simulink model "omnimorph_controller_FL"  (R2023b)
settings: Solver=ode1  StartTime=0.0  StopTime=inf  FixedStep=config.simVar.timeStep  RelTol=1e-3
libraries: genomix x5, robotcorelib x4
settings Model: Creator=amr  LastModifiedBy=fiore
settings DataIOCC: ReturnWorkspaceOutputs=off
settings OptimizationCC: ReuseModelBlockBuffer=off
settings DebuggingCC: UnconnectedInputMsg=warning  UnconnectedOutputMsg=warning  UnconnectedLineMsg=warning  UnderSpecifiedDimensionMsg=warning
settings ModelReferenceCC: EnableRefExpFcnMdlSchedulingChecks=on
settings RTWCC: DLArmComputeVersion=19.05

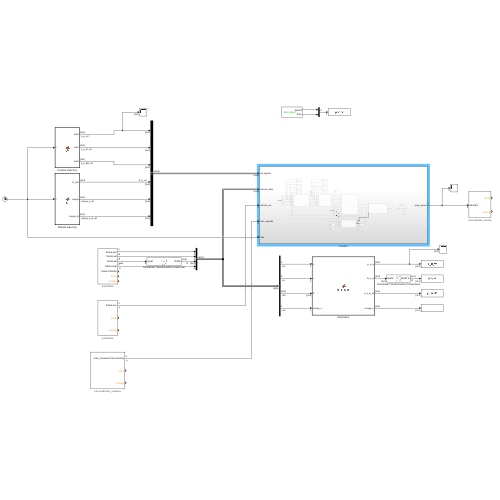
[thumbnail: Simulink's stored preview of the top-level diagram]
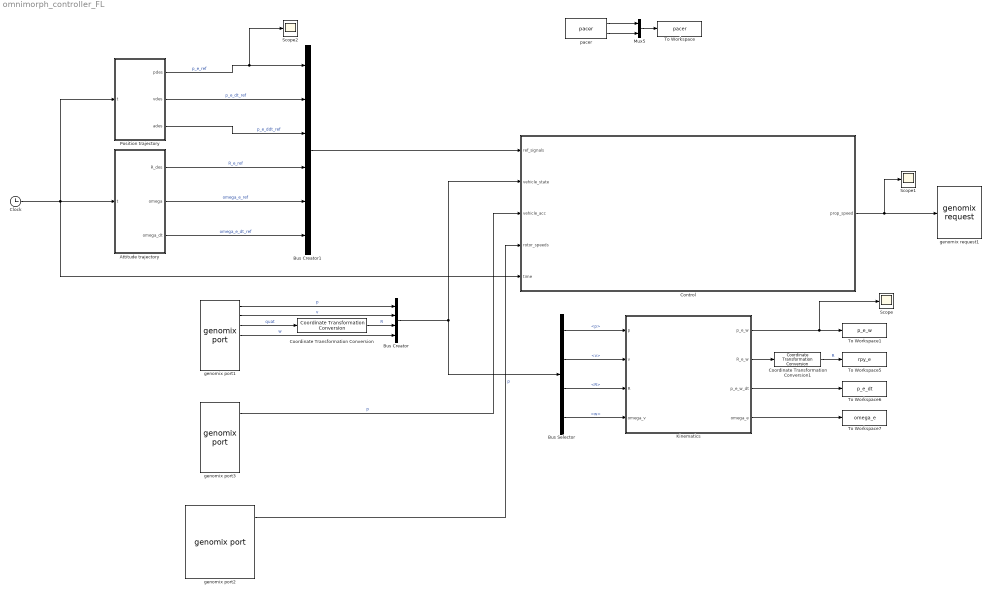
== system omnimorph_controller_FL ==
  Attitude trajectory : MATLAB Function  TreatAsAtomicUnit=on
  Bus Creator : BusCreator  Inputs=4
  Bus Creator1 : BusCreator  Inputs=6
  Bus Selector : BusSelector  OutputSignals=p,v,R,w
  Clock : Clock
  Control : Subsystem
  Coordinate Transformation Conversion : robotcorelib/Coordinate Transformation Conversion  InputRepresentation=Quaternion  InputEulerSequence=ZYX  ShowTrVecInputPort=on  OutputRepresentation=Rotation Matrix  OutputEulerSequence=ZYX  ShowTrVecOutputPort=on  SimulateUsing=Interpreted execution
  Coordinate Transformation Conversion1 : robotcorelib/Coordinate Transformation Conversion  InputRepresentation=Rotation Matrix  InputEulerSequence=ZYX  ShowTrVecInputPort=on  OutputRepresentation=Euler Angles  OutputEulerSequence=ZYX  ShowTrVecOutputPort=on  SimulateUsing=Interpreted execution
  Kinematics : MATLAB Function  TreatAsAtomicUnit=on
  Mux5 : Mux  Inputs=2
  Position trajectory : MATLAB Function  TreatAsAtomicUnit=on
  Scope : Scope
  Scope1 : Scope
  Scope2 : Scope
  To Workspace : ToWorkspace  VariableName=pacer  SaveFormat=Timeseries  SampleTime=-1
  To Workspace1 : ToWorkspace  VariableName=p_e_w  SampleTime=-1
  To Workspace5 : ToWorkspace  VariableName=rpy_e  SampleTime=-1
  To Workspace6 : ToWorkspace  VariableName=p_e_dt  SampleTime=-1
  To Workspace7 : ToWorkspace  VariableName=omega_e  SampleTime=-1
  genomix port1 : genomix/genomix port  host=localhost  component=pom  port=frame  subport=robot  sigtype=value  timetype=periodic  period=config.simVar.timeStep  siglist="[{\"name\":\"frame.pos\",\"type\":\"value\",\"size\":3},{\"name\":\"frame.vel\",\"type\":\"value\",\"size\":3},{\"name\":\"frame.att\",\"type\":\"value\",\"size\":4},{\"name\":\"frame.avel\",\"type\":\"value\",\"size\":3},{\"name\":\"frame.intrinsic\",\"type\":\"value\",\"size\":1}]"
      settings: AttributesFormatString=pom/frame
  genomix port2 : genomix/genomix port  host=localhost  component=rotorcraft  port=rotor_measure  sigtype=value  timetype=periodic  period=config.simVar.timeStep  siglist="[{\"name\":\"rotor_measure.rotor.velocity\",\"type\":\"value\",\"size\":8}]"
      settings: AttributesFormatString=rotorcraft/rotor_measure
  genomix port3 : genomix/genomix port  host=localhost  component=pom  port=frame  subport=robot  sigtype=value  timetype=periodic  period=config.simVar.timeStep  siglist="[{\"name\":\"frame.acc\",\"type\":\"value\",\"size\":3}]"
      settings: AttributesFormatString=pom/frame
  genomix request1 : genomix/genomix request  host=localhost  component=rotorcraft  port=set_velocity  sigtype=value  timetype=periodic  period=config.simVar.timeStep  siglist="[{\"name\":\"desired\",\"type\":\"value\",\"size\":8}]"
      settings: AttributesFormatString=rotorcraft/set_velocity
  pacer : genomix/pacer  Priority=0  catchup=off
  wires:
  genomix port1/1 -> Bus Creator/1  "p"
  genomix port1/2 -> Bus Creator/2  "v"
  genomix port1/4 -> Bus Creator/4  "w"
  genomix port1/3 -> Coordinate Transformation Conversion/1  "quat"
  Coordinate Transformation Conversion/1 -> Bus Creator/3  "R"
  Bus Creator/1 -> Bus Selector/1, Control/2(vehicle_state)
  Control/1(prop_speed) -> Scope1/1, genomix request1/1
  pacer/2 -> Mux5/2
  pacer/1 -> Mux5/1
  Mux5/1 -> To Workspace/1
  genomix port3/1 -> Control/3(vehicle_acc)  "p"
  genomix port2/1 -> Control/4(rotor_speeds)  "p"
  Kinematics/1(p_e_w) -> Scope/1, To Workspace1/1
  Kinematics/3(p_e_w_dt) -> To Workspace6/1
  Kinematics/4(omega_e) -> To Workspace7/1
  Coordinate Transformation Conversion1/1 -> To Workspace5/1  "R"
  Kinematics/2(R_e_w) -> Coordinate Transformation Conversion1/1
  Bus Selector/1 -> Kinematics/1(p)  "<p>"
  Bus Selector/2 -> Kinematics/2(v)  "<v>"
  Bus Selector/3 -> Kinematics/3(R)  "<R>"
  Bus Selector/4 -> Kinematics/4(omega_v)  "<w>"
  Attitude trajectory/1(R_des) -> Bus Creator1/4  "R_e_ref"
  Attitude trajectory/2(omega) -> Bus Creator1/5  "omega_e_ref"
  Position trajectory/3(ades) -> Bus Creator1/3  "p_e_ddt_ref"
  Clock/1 -> Control/5(time), Position trajectory/1(t), Attitude trajectory/1(t)
  Bus Creator1/1 -> Control/1(ref_signals)
  Position trajectory/2(vdes) -> Bus Creator1/2  "p_e_dt_ref"
  Attitude trajectory/3(omega_dt) -> Bus Creator1/6  "omega_e_dt_ref"
  Position trajectory/1(pdes) -> Scope2/1, Bus Creator1/1  "p_e_ref"

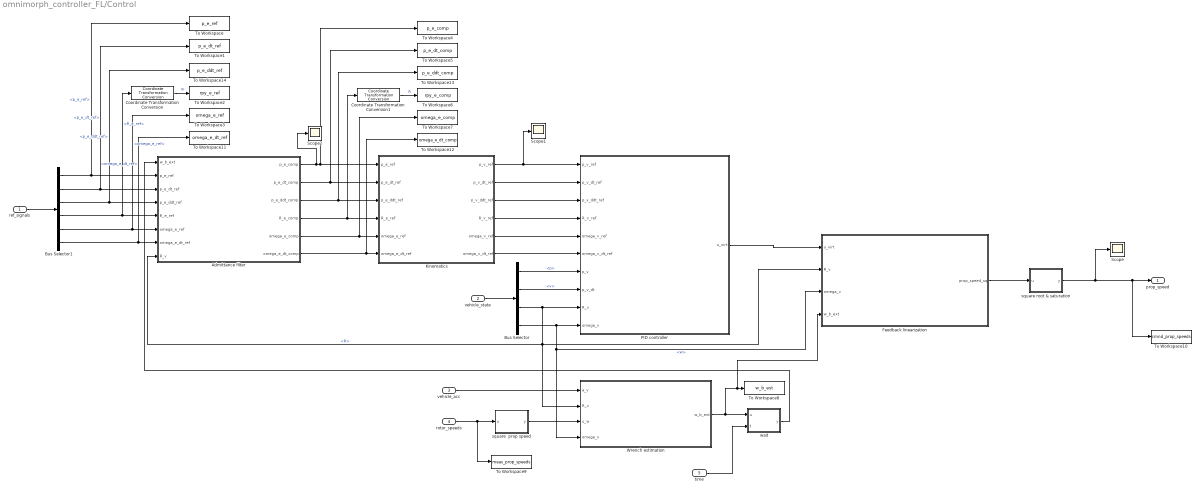
== system omnimorph_controller_FL/Control ==
  ref_signals : Inport
  vehicle_state : Inport  Port=2
  vehicle_acc : Inport  Port=3
  rotor_speeds : Inport  Port=4
  time : Inport  Port=5
  Admittance filter : Subsystem
  Bus Selector : BusSelector  OutputSignals=p,v,R,w
  Bus Selector1 : BusSelector  OutputSignals=p_e_ref,p_e_dt_ref,p_e_ddt_ref,R_e_ref,omega_e_ref,omega_e_dt_ref
  Coordinate Transformation Conversion : robotcorelib/Coordinate Transformation Conversion  InputRepresentation=Rotation Matrix  InputEulerSequence=ZYX  ShowTrVecInputPort=on  OutputRepresentation=Euler Angles  OutputEulerSequence=ZYX  ShowTrVecOutputPort=on  SimulateUsing=Interpreted execution
  Coordinate Transformation Conversion1 : robotcorelib/Coordinate Transformation Conversion  InputRepresentation=Rotation Matrix  InputEulerSequence=ZYX  ShowTrVecInputPort=on  OutputRepresentation=Euler Angles  OutputEulerSequence=ZYX  ShowTrVecOutputPort=on  SimulateUsing=Interpreted execution
  Feedback linearization : MATLAB Function  TreatAsAtomicUnit=on
  Kinematics : MATLAB Function  TreatAsAtomicUnit=on
  PID controller : MATLAB Function  TreatAsAtomicUnit=on
  Scope : Scope
  Scope1 : Scope
  Scope2 : Scope
  To Workspace : ToWorkspace  VariableName=p_e_ref  SampleTime=-1
  To Workspace1 : ToWorkspace  VariableName=p_e_dt_ref  SampleTime=-1
  To Workspace10 : ToWorkspace  VariableName=cmnd_prop_speeds  SampleTime=-1
  To Workspace11 : ToWorkspace  VariableName=omega_e_dt_ref  SampleTime=-1
  To Workspace12 : ToWorkspace  VariableName=omega_e_dt_comp  SampleTime=-1
  To Workspace13 : ToWorkspace  VariableName=p_e_ddt_comp  SampleTime=-1
  To Workspace14 : ToWorkspace  VariableName=p_e_ddt_ref  SampleTime=-1
  To Workspace2 : ToWorkspace  VariableName=rpy_e_ref  SampleTime=-1
  To Workspace3 : ToWorkspace  VariableName=omega_e_ref  SampleTime=-1
  To Workspace4 : ToWorkspace  VariableName=p_e_comp  SampleTime=-1
  To Workspace5 : ToWorkspace  VariableName=p_e_dt_comp  SampleTime=-1
  To Workspace6 : ToWorkspace  VariableName=rpy_e_comp  SampleTime=-1
  To Workspace7 : ToWorkspace  VariableName=omega_e_comp  SampleTime=-1
  To Workspace8 : ToWorkspace  VariableName=w_b_est  SampleTime=-1
  To Workspace9 : ToWorkspace  VariableName=meas_prop_speeds  SampleTime=-1
  Wrench estimation : Subsystem
  square  prop speed : MATLAB Function  TreatAsAtomicUnit=on
  square root & saturation : MATLAB Function  TreatAsAtomicUnit=on
  wait : MATLAB Function  TreatAsAtomicUnit=on
  prop_speed : Outport
  wires:
  PID controller/1(u_virt) -> Feedback linearization/1(u_virt)
  Bus Selector/4 -> PID controller/10(omega_v), Wrench estimation/4(omega_v), Feedback linearization/3(omega_v)  "<w>"
  ref_signals/1 -> Bus Selector1/1
  square root & saturation/1(y) -> Scope/1, prop_speed/1, To Workspace10/1
  Admittance filter/1(p_e_comp) -> Scope2/1, To Workspace4/1, Kinematics/1(p_e_ref)
  Admittance filter/2(p_e_dt_comp) -> To Workspace5/1, Kinematics/2(p_e_dt_ref)
  Admittance filter/3(p_e_ddt_comp) -> To Workspace13/1, Kinematics/3(p_e_ddt_ref)
  Admittance filter/6(omega_e_dt_comp) -> To Workspace12/1, Kinematics/6(omega_e_dt_ref)
  Bus Selector1/6 -> To Workspace11/1, Admittance filter/7(omega_e_dt_ref)  "<omega_e_dt_ref>"
  Bus Selector1/5 -> To Workspace3/1, Admittance filter/6(omega_e_ref)  "<omega_e_ref>"
  Bus Selector1/4 -> Admittance filter/5(R_e_ref), Coordinate Transformation Conversion/1  "<R_e_ref>"
  Bus Selector1/3 -> To Workspace14/1, Admittance filter/4(p_e_ddt_ref)  "<p_e_ddt_ref>"
  Bus Selector1/2 -> To Workspace1/1, Admittance filter/3(p_e_dt_ref)  "<p_e_dt_ref>"
  Admittance filter/4(R_e_comp) -> Kinematics/4(R_e_ref), Coordinate Transformation Conversion1/1
  Kinematics/1(p_v_ref) -> Scope1/1, PID controller/1(p_v_ref)
  Kinematics/2(p_v_dt_ref) -> PID controller/2(p_v_dt_ref)
  Kinematics/3(p_v_ddt_ref) -> PID controller/3(p_v_ddt_ref)
  Kinematics/5(omega_v_ref) -> PID controller/5(omega_v_ref)
  Kinematics/6(omega_v_dt_ref) -> PID controller/6(omega_v_dt_ref)
  Kinematics/4(R_v_ref) -> PID controller/4(R_v_ref)
  Admittance filter/5(omega_e_comp) -> Kinematics/5(omega_e_ref), To Workspace7/1
  Bus Selector/1 -> PID controller/7(p_v)  "<p>"
  Bus Selector/2 -> PID controller/8(p_v_dt)  "<v>"
  Bus Selector/3 -> Wrench estimation/2(R_v), Admittance filter/8(R_v), Feedback linearization/2(R_v), PID controller/9(R_v)  "<R>"
  Feedback linearization/1(prop_speed_sq) -> square root & saturation/1(u)
  vehicle_state/1 -> Bus Selector/1
  vehicle_acc/1 -> Wrench estimation/1(a_v)
  rotor_speeds/1 -> To Workspace9/1, square  prop speed/1(u)
  square  prop speed/1(y) -> Wrench estimation/3(u_w)
  wait/1(y) -> Admittance filter/1(w_b_ext)
  time/1 -> wait/2(t)
  Bus Selector1/1 -> To Workspace/1, Admittance filter/2(p_e_ref)  "<p_e_ref>"
  Wrench estimation/1(w_b_ext) -> Feedback linearization/4(w_b_ext), To Workspace8/1, wait/1(u)
  Coordinate Transformation Conversion/1 -> To Workspace2/1  "R"
  Coordinate Transformation Conversion1/1 -> To Workspace6/1  "R"

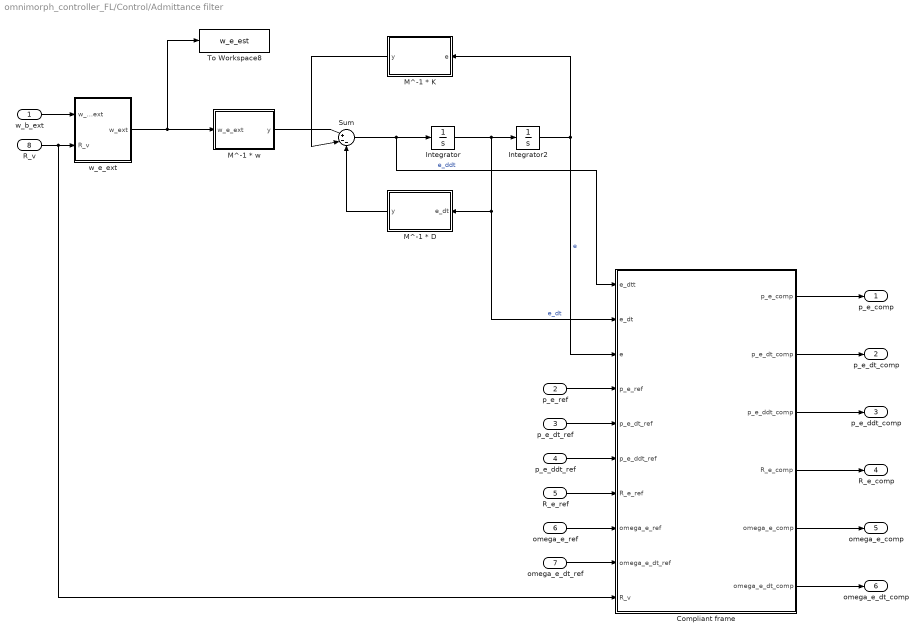
== system omnimorph_controller_FL/Control/Admittance filter ==
  w_b_ext : Inport
  p_e_ref : Inport  Port=2
  p_e_dt_ref : Inport  Port=3
  p_e_ddt_ref : Inport  Port=4
  R_e_ref : Inport  Port=5
  omega_e_ref : Inport  Port=6
  omega_e_dt_ref : Inport  Port=7
  R_v : Inport  Port=8
  Compliant frame : MATLAB Function  TreatAsAtomicUnit=on
  Integrator : Integrator
  Integrator2 : Integrator
  M^-1 * D : MATLAB Function  TreatAsAtomicUnit=on
  M^-1 * K : MATLAB Function  TreatAsAtomicUnit=on
  M^-1 * w : MATLAB Function  TreatAsAtomicUnit=on
  Sum : Sum  Inputs=|+--
  To Workspace8 : ToWorkspace  VariableName=w_e_est  SampleTime=-1
  w_e_ext : MATLAB Function  TreatAsAtomicUnit=on
  p_e_comp : Outport
  p_e_dt_comp : Outport  Port=2
  p_e_ddt_comp : Outport  Port=3
  R_e_comp : Outport  Port=4
  omega_e_comp : Outport  Port=5
  omega_e_dt_comp : Outport  Port=6
  wires:
  Integrator/1 -> Compliant frame/2(e_dt), M^-1 * D/1(e_dt), Integrator2/1  "e_dt"
  Sum/1 -> Compliant frame/1(e_dtt), Integrator/1  "e_ddt"
  M^-1 * K/1(y) -> Sum/2
  Integrator2/1 -> Compliant frame/3(e), M^-1 * K/1(e)  "e"
  M^-1 * D/1(y) -> Sum/3
  p_e_ref/1 -> Compliant frame/4(p_e_ref)
  p_e_dt_ref/1 -> Compliant frame/5(p_e_dt_ref)
  p_e_ddt_ref/1 -> Compliant frame/6(p_e_ddt_ref)
  R_e_ref/1 -> Compliant frame/7(R_e_ref)
  omega_e_ref/1 -> Compliant frame/8(omega_e_ref)
  omega_e_dt_ref/1 -> Compliant frame/9(omega_e_dt_ref)
  Compliant frame/6(omega_e_dt_comp) -> omega_e_dt_comp/1
  Compliant frame/5(omega_e_comp) -> omega_e_comp/1
  Compliant frame/4(R_e_comp) -> R_e_comp/1
  Compliant frame/3(p_e_ddt_comp) -> p_e_ddt_comp/1
  Compliant frame/2(p_e_dt_comp) -> p_e_dt_comp/1
  Compliant frame/1(p_e_comp) -> p_e_comp/1
  M^-1 * w/1(y) -> Sum/1
  w_b_ext/1 -> w_e_ext/1(w_b_ext)
  R_v/1 -> Compliant frame/10(R_v), w_e_ext/2(R_v)
  w_e_ext/1(w_ext) -> To Workspace8/1, M^-1 * w/1(w_e_ext)

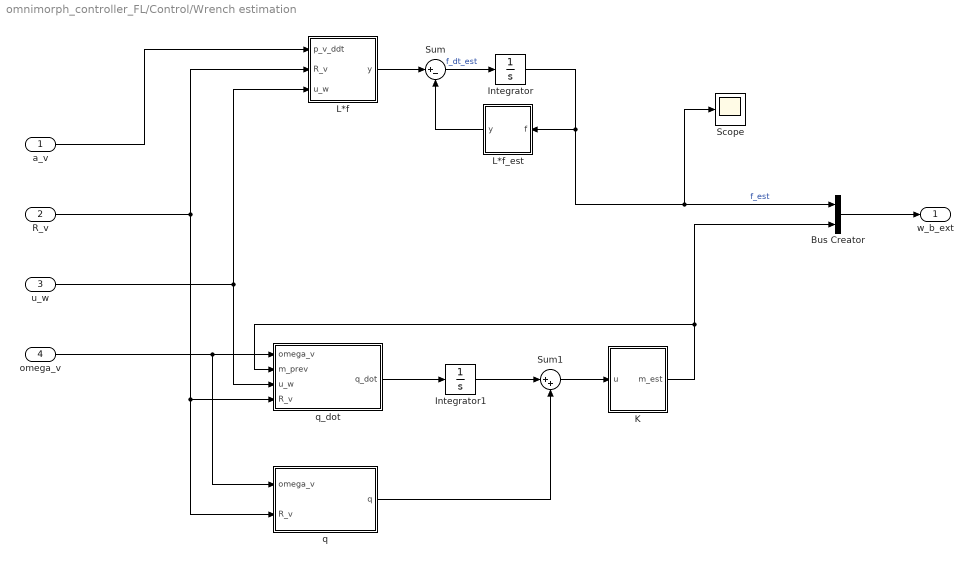
== system omnimorph_controller_FL/Control/Wrench estimation ==
  a_v : Inport
  R_v : Inport  Port=2
  u_w : Inport  Port=3
  omega_v : Inport  Port=4
  Bus Creator : BusCreator  Inputs=2
  Integrator : Integrator
  Integrator1 : Integrator
  K : MATLAB Function  TreatAsAtomicUnit=on
  L*f : MATLAB Function  TreatAsAtomicUnit=on
  L*f_est : MATLAB Function  TreatAsAtomicUnit=on
  Scope : Scope
  Sum : Sum  Inputs=|+-
  Sum1 : Sum  Inputs=|++
  q : MATLAB Function  TreatAsAtomicUnit=on
  q_dot : MATLAB Function  TreatAsAtomicUnit=on
  w_b_ext : Outport
  wires:
  Sum/1 -> Integrator/1  "f_dt_est"
  Integrator/1 -> Scope/1, Bus Creator/1, L*f_est/1(f)  "f_est"
  L*f_est/1(y) -> Sum/2
  L*f/1(y) -> Sum/1
  R_v/1 -> q/2(R_v), q_dot/4(R_v), L*f/2(R_v)
  u_w/1 -> q_dot/3(u_w), L*f/3(u_w)
  omega_v/1 -> q/1(omega_v), q_dot/1(omega_v)
  a_v/1 -> L*f/1(p_v_ddt)
  Integrator1/1 -> Sum1/1
  q/1(q) -> Sum1/2
  Sum1/1 -> K/1(u)
  q_dot/1(q_dot) -> Integrator1/1
  Bus Creator/1 -> w_b_ext/1
  K/1(m_est) -> Bus Creator/2, q_dot/2(m_prev)

== matlab function omnimorph_controller_FL/Control/Admittance filter/M^-1 * D ==
  data: e_dt input; y output; config parameter
function y = fcn(e_dt,config)

D = config.conrtolParams.admitFilt.virtDamp;
M = config.conrtolParams.admitFilt.virtMass;
%invM = diag([1/M(1,1);1/M(2,2);1/M(3,3)]);
invM = diag([1/M(1,1);1/M(2,2);1/M(3,3);1/M(4,4);1/M(5,5);1/M(6,6)]);

y = invM*D*e_dt;

end

== matlab function omnimorph_controller_FL/Control/Admittance filter/Compliant frame ==
  data: e_dtt input; e_dt input; e input; p_e_ref input; p_e_dt_ref input; p_e_ddt_ref input; R_e_ref input; omega_e_ref input; omega_e_dt_ref input; R_v input; p_e_comp output; config parameter; p_e_dt_comp output; p_e_ddt_comp output; R_e_comp output; omega_e_comp output; omega_e_dt_comp output
function [p_e_comp,p_e_dt_comp,p_e_ddt_comp,R_e_comp,omega_e_comp,omega_e_dt_comp] = fcn(e_dtt,e_dt,e,p_e_ref,p_e_dt_ref,p_e_ddt_ref, ...
                                                                                 R_e_ref,omega_e_ref,omega_e_dt_ref,R_v,config)
p_e_comp = p_e_ref + e(1:3);
p_e_dt_comp = p_e_dt_ref + e_dt(1:3);
p_e_ddt_comp = p_e_ddt_ref + e_dtt(1:3);

R_e_comp = (skewMat(e(4:6)) + eye(3))*R_e_ref;
omega_e_comp = omega_e_ref + e_dt(4:6);
omega_e_dt_comp = omega_e_dt_ref + e_dtt(4:6);
end

== matlab function omnimorph_controller_FL/Control/Admittance filter/M^-1 * w ==
  data: w_e_ext input; y output; config parameter
function y = fcn(w_e_ext,config)

M = config.conrtolParams.admitFilt.virtMass;
invM = diag([1/M(1,1);1/M(2,2);1/M(3,3);1/M(4,4);1/M(5,5);1/M(6,6)]);

y = invM*w_e_ext;

end

== matlab function omnimorph_controller_FL/Kinematics ==
  settings: updateMethod=DISCRETE
  data: p input; v input; R input; omega_v input; config parameter; p_e_w output; R_e_w output; p_e_w_dt output; omega_e output
function [p_e_w,R_e_w,p_e_w_dt,omega_e] = kinematic(p,v,R,omega_v,config)

p_e = config.uavParams.endEffector.p_e;
R_e = config.uavParams.endEffector.R_e;

p_e_w = p + R*p_e;
R_e_w = R*R_e;

omega_e = omega_v;
p_e_w_dt = v + R*skewMat(omega_v)*p_e;

end

== matlab function omnimorph_controller_FL/Control/Kinematics ==
  settings: updateMethod=DISCRETE
  data: p_e_ref input; p_e_dt_ref input; p_e_ddt_ref input; R_e_ref input; omega_e_ref input; omega_e_dt_ref input; config parameter; p_v_ref output; p_v_dt_ref output; p_v_ddt_ref output; R_v_ref output; omega_v_ref output; omega_v_dt_ref output
function [p_v_ref,p_v_dt_ref,p_v_ddt_ref,R_v_ref,omega_v_ref,omega_v_dt_ref] = kinematic(p_e_ref,p_e_dt_ref,p_e_ddt_ref,R_e_ref,omega_e_ref,omega_e_dt_ref,config)

p_e = config.uavParams.endEffector.p_e ;
R_e = config.uavParams.endEffector.R_e;

% R_v_ref = R_e_ref*R_e.';
% p_v_ref = p_e_ref - R_v_ref*p_e;
% 
% omega_v_ref = omega_e_ref;
% p_v_dt_ref = p_e_dt_ref - R_v_ref*skewMat(omega_v_ref)*p_e;
% 
% omega_v_dt_ref = omega_e_dt_ref;
% p_v_ddt_ref = p_e_ddt_ref - R_v_ref*skewMat(omega_v_dt_ref)*p_e - R_v_ref*skewMat(omega_v_ref)^2 *p_e;

R_v_ref = R_e_ref*R_e.';
p_v_ref = p_e_ref - R_v_ref*p_e;

omega_v_ref = omega_e_ref;
p_v_dt_ref = p_e_dt_ref - skewMat(omega_v_ref)*R_v_ref*p_e;

omega_v_dt_ref = omega_e_dt_ref;
p_v_ddt_ref = p_e_ddt_ref - skewMat(omega_v_dt_ref)*R_v_ref*p_e - skewMat(omega_v_ref)^2 *R_v_ref*p_e;
end

== matlab function omnimorph_controller_FL/Control/Wrench estimation/L*f_est ==
  settings: updateMethod=DISCRETE
  data: f input; config parameter; y output
function y = fcn(f,config)

L = config.conrtolParams.wrenchObs.gains(1:3,1:3);
y = L*f;

end

== matlab function omnimorph_controller_FL/Control/Wrench estimation/L*f ==
  settings: updateMethod=DISCRETE
  data: p_v_ddt input; R_v input; u_w input; config parameter; y output
function y = fcn(p_v_ddt,R_v,u_w,config)

L = config.conrtolParams.wrenchObs.gains(1:3,1:3);
m = config.uavParams.mass;
g = config.gravity;
A = config.uavParams.wrenchMap;

f = m*p_v_ddt + m*g*[0;0;1] - R_v*A(1:3,:)*u_w;

y = L*f;

end

== matlab function omnimorph_controller_FL/Control/Wrench estimation/q_dot ==
  settings: updateMethod=DISCRETE
  data: omega_v input; m_prev input; u_w input; R_v input; config parameter; q_dot output size=[3 1]
function q_dot = fcn(omega_v,m_prev,u_w,R_v,config)

A = config.uavParams.wrenchMap;
J = config.uavParams.inertia;
omega_v_b = R_v'*omega_v; % Body frame angular velocity

q_dot = cross(omega_v_b,(J*omega_v_b)) - A(4:6,:)*u_w - m_prev;

end

== matlab function omnimorph_controller_FL/Control/Wrench estimation/q ==
  settings: updateMethod=DISCRETE
  data: omega_v input; R_v input; config parameter; q output
function q = fcn(omega_v,R_v,config)

J = config.uavParams.inertia;
omega_v_b = R_v'*omega_v; % Body frame angular velocity

% Assuming initial angular velocity is zero
q = J*omega_v_b;

end

== matlab function omnimorph_controller_FL/Control/Wrench estimation/K ==
  settings: updateMethod=DISCRETE
  data: u input; config parameter; m_est output
function m_est = fcn(u,config)

K = config.conrtolParams.wrenchObs.gains(4:6,4:6);
m_est = K*u;

end

== matlab function omnimorph_controller_FL/Control/Admittance filter/w_e_ext ==
  data: w_b_ext input; R_v input; w_ext output; config parameter
function w_ext = fcn(w_b_ext,R_v,config)

p_e = config.uavParams.endEffector.p_e;

H =  [eye(3),zeros(3);skewMat(R_v*p_e),eye(3)];
w_ext = H\[w_b_ext(1:3);R_v*w_b_ext(4:6)];

end

== matlab function omnimorph_controller_FL/Control/square root & saturation ==
  data: u input; y output; config parameter
function y = fcn(u,config)   
    prop_max = config.uavParams.maxPropSpeed;
    prop_min = config.uavParams.minPropSpeed;

    y = sign(u) .* sqrt(abs(u));
    y = min(y, prop_max); % Clip positive values
    y = max(y, prop_min); % Clip negative values
end

== matlab function omnimorph_controller_FL/Position trajectory ==
  data: t input; pdes output; vdes output; ades output; config parameter
function [pdes,vdes,ades] = fcn(t,config)

r = config.trajParams.radius;
f = config.trajParams.frequency;
z = 1;

% Circular trajectory
if t<2
   [pdes,vdes,ades] = circ_traj(t,0.5*t,f,0.5*t);
   vdes(3) = 0.5;
else
   [pdes,vdes,ades] = circ_traj(t,r,f,z);
end

% Peg-in-hole task
% if t<2
%     pdes = [0;0;0.5*t];
%     vdes = [0;0;0.5];
%     ades = [0;0;0];
% elseif t>=2 && t<16.5
%     pdes = [0.1*(t-2);0;0.99];
%     vdes = [0.1;0;0];
%     ades = [0;0;0];
% else
%     pdes = [(0.1*(16.5-2))-0.1*(t-16.5);0;0.99];
%     vdes = [-0.1;0;0];
%     ades = [0;0;0];    
% end

% Sliding task
%if t<2
%    pdes = [0;0;0.5*t];
%    vdes = [0;0;0.5];
%    ades = [0;0;0];
%elseif t>=2 && t<14
%   pdes = [0.1*(t-2);0;1];
%   vdes = [0.1;0;0];
%   ades = [0;0;0]; 
%else
%   pdes = [1.2;0;1+0.1*(t-14)];
%   vdes = [0;0;0.1];
%   ades = [0;0;0]; 
%end

end

== matlab function omnimorph_controller_FL/Control/PID controller ==
  settings: updateMethod=DISCRETE
  data: p_v_ref input; p_v_dt_ref input; p_v_ddt_ref input; R_v_ref input; omega_v_ref input; omega_v_dt_ref input; p_v input; p_v_dt input; R_v input; omega_v input; config parameter; u_virt output
function u_virt  = PIDPlus(p_v_ref,p_v_dt_ref,p_v_ddt_ref, ...
                                          R_v_ref,omega_v_ref,omega_v_dt_ref,...
                                          p_v,p_v_dt,...
                                          R_v,omega_v,config)

persistent eI_prev

if isempty(eI_prev)
    eI_prev = zeros(6,1);
end

%% initializations
u_virt = zeros(6,1);

Kp = config.conrtolParams.gainsPID.Kp;
Kv = config.conrtolParams.gainsPID.Kv;
KR = config.conrtolParams.gainsPID.KR;
Kw = config.conrtolParams.gainsPID.Kw;
KI_p = config.conrtolParams.gainsPID.KI_p;

dt = config.simVar.timeStep;

%omega_v = R_v'*omega_v;

%% error signal computations 
ep =  p_v_ref - p_v;
ev = p_v_dt_ref - p_v_dt;
eI_p = eI_prev(1:3) + ep*dt;

eR = vmap(R_v_ref,R_v);
%ew = R_v.' * (omega_v_ref - omega_v);

ew = omega_v_ref - (R_v.')*R_v_ref*omega_v;
eI_R = eI_prev(4:6) + eR*dt;

eI_prev = [eI_p; eI_R];

%% compute u_virt
u_virt(1:3) = p_v_ddt_ref + Kv*ev + Kp*ep + KI_p*eI_p; 
u_virt(4:6) = omega_v_dt_ref + Kw*ew + KR*eR; 
end

== matlab function omnimorph_controller_FL/Control/Feedback linearization ==
  settings: updateMethod=DISCRETE
  data: u_virt input size=[6, 1]; prop_speed_sq output size=[8,1]; R_v input size=[3, 3]; omega_v input; w_b_ext input; config parameter
function prop_speed_sq = cntrl_FL(u_virt,R_v,omega_v,w_b_ext,config)

% initializations
m = config.uavParams.mass; % uav mass
J = config.uavParams.inertia;%3x3 diag. uav Inertia mat.
A = config.uavParams.wrenchMap;
g = config.gravity;
omega_v = R_v'*omega_v;% Body frame angular velocity

J_inv = diag([1/J(1,1),1/J(2,2),1/J(3,3)]);
invInertia_mat = [eye(3)*(1/m), zeros(3); zeros(3),J_inv];
A_bar = invInertia_mat*[R_v, zeros(3); zeros(3), eye(3)]*A;
bias_forces = -[g*[0;0;1];J_inv*cross(omega_v,(J*omega_v))];
w_b = invInertia_mat*w_b_ext;

% feedback linearization
prop_speed_sq = pinv(A_bar)*( - bias_forces + u_virt - w_b);

end

% function prop_speed_sq = cntrl_FL(u_virt,R_v,omega_v,config,t,w_cur)
% % initializations
% m = config.uavParams.mass; % uav mass
% J = config.uavParams.inertia;%3x3 diag. uav Inertia mat.
% A = config.uavParams.wrenchMap;
% g = config.gravity;
% omega_v = R_v'*omega_v;
% J_inv = diag([1/J(1,1),1/J(2,2),1/J(3,3)]);
% invInertia_mat = [eye(3)*(1/m), zeros(3); zeros(3),J_inv];
% A_bar = invInertia_mat*[R_v, zeros(3); zeros(3), eye(3)]*A;
% bias_forces = -[g*[0;0;1];J_inv*cross(omega_v,(J*omega_v))];
% 
% % feedback linearization
% %prop_speed_sq = wrench2u_hybrid(A_bar, (-bias_forces + u_virt), 8);
% 
% lb=30*30; ub=220*220;
% prop_speed_sq = zeros(8,1);  % force fixed size
% 
% persistent y_prev u_prev t_miqp k_miqp y_prev_measured
% 
% if isempty(y_prev)
%     y_prev = ones(8,1);   
% else
%     y_prev = y_prev(:); 
% end
% if isempty(u_prev)
%     u_prev = 50*ones(8,1);
% else
%     u_prev = u_prev(:);
% end
% if isempty(y_prev_measured)
%     y_prev_measured = double(sign(w_cur) > 0);   
% else
%     y_prev_measured = y_prev_measured(:);
% end
% if isempty(t_miqp)
%     t_miqp = 0;  
% end
% if isempty(k_miqp)
%     k_miqp = 0;   
% end
% w_cur_zero_idx=find(w_cur==0);
% y_measured=[];
% if isempty(w_cur_zero_idx)
%     y_measured=double(sign(w_cur) > 0);
% else
%     y_measured=double(sign(w_cur) > 0);
%     y_measured(w_cur_zero_idx)=y_prev_measured(w_cur_zero_idx);
% end
%  y_prev_measured(:)=y_measured;
%  u_pinv = pinv(A_bar)*(-bias_forces + u_virt);
%  pinv_feasible = all(abs(u_pinv) >= lb & abs(u_pinv) <= ub);
%  near_lb_idx = find(y_prev~=y_prev_measured);
%  all_measu=all(y_prev==y_prev_measured & abs(w_cur) >= lb);
%  Q=eye(8,8);
%  w=(-bias_forces + u_virt);
%  A=A_bar;
%  if pinv_feasible && all_measu
%      % Directly accept the pseudoinverse solution
%      prop_speed_sq(:) = u_pinv(:);
%      u_prev(:) = u_pinv(:);
%      sgn = sign(u_pinv);
%      y_prev = double(sgn > 0);
%  else
%      tic;
%      % --- Identify indices near lower bound ---
%      if ~isempty(near_lb_idx)
%          % Fix corresponding y values to previous pattern
%          y_fixed = NaN(size(y_prev));
%          y_fixed(near_lb_idx) = y_prev(near_lb_idx);
% 
%          % Objective 1: 0.5*u'*Q*u, equality constraint ON
%          objective.Q = Q;
%          objective.f = zeros(size(Q,1),1);
%          Aeq_on = 1;
%          [u_best, y_best, cost_best, flag] = solve_miqp_bb_stack_2( ...
%              w, A, Q, lb, ub, u_prev, y_prev, y_fixed, objective, Aeq_on);
%      else
%          % No propeller near lower bound → solve full MIQP with all y free
%          y_fixed = NaN(size(y_prev));
%          objective.Q = Q;
%          objective.f = zeros(size(Q,1),1);
%          Aeq_on = 1;
%          [u_best, y_best, cost_best, flag] = solve_miqp_bb_stack_2( ...
%              w, A, Q, lb, ub, u_prev, y_prev, y_fixed, objective, Aeq_on);
%     end
% 
%      % --- First fallback: relaxed objective if infeasible ---
%      if flag ~= 1
%          disp('First MIQP infeasible, trying relaxed objective.');
%          objective.Q = Q + A'*A;
%          objective.f = -A'*w;  
%          Aeq_on = 0;     % remove equality constraint
%          [u_best, y_best, cost_best, flag] = solve_miqp_bb_stack_2( ...
%              w, A, Q, lb, ub, u_prev, y_prev, y_fixed, objective, Aeq_on);
%          if flag==1
%              disp('trying relaxed objective..success');
%          end
%      end
% 
%      % --- Second fallback: plain QP with equality ---
%      if flag ~= 1
%          disp('Second MIQP infeasible, fallback QP with equality.');
%          H = Q;
%          f = zeros(size(Q,1),1);
%          Aeq = A;
%          beq = w;
%          lb_u = -ub * ones(8,1);
%          ub_u =  ub * ones(8,1);
%          [u_qp, ~, exitflag_qp] = quadprog(H, f, [], [], Aeq, beq, lb_u, ub_u, u_prev, ...
%              optimoptions('quadprog','Algorithm','active-set','Display','off'));
%          if exitflag_qp == 1
%              u_best = u_qp;
%              sgn = sign(u_best);
%              y_prev(:) = double(sgn>0);
%              flag = 1;
%          else
%              disp('QP also infeasible, using previous u.');
%              u_best = u_prev;
%              y_best = y_prev;
%          end
%      end
% 
%      % --- Store final results ---
%      if flag == 1
%         u_prev(:) = u_best(:);
%          y_prev(:) = y_best(:);
%          prop_speed_sq(:) = u_best(:);
%      else
%          disp('All fallback stages infeasible. Keeping previous control.');
%          prop_speed_sq(:) = u_prev(:);
%      end
% 
%      % Timing
%     t_miqp = t_miqp + toc;
%     k_miqp = k_miqp + 1;
%  end
% 
%  if t == 20
%      disp(t_miqp / k_miqp);
%  end
% end

== matlab function omnimorph_controller_FL/Control/square  prop speed ==
  data: u input; y output
function y = fcn(u)
    y = sign(u) .* (abs(u).^2);
end

== matlab function omnimorph_controller_FL/Control/Admittance filter/M^-1 * K ==
  data: e input; y output; config parameter
function y = fcn(e,config)

K = config.conrtolParams.admitFilt.virtStiff;
M = config.conrtolParams.admitFilt.virtMass;
%invM = diag([1/M(1,1);1/M(2,2);1/M(3,3)]);
invM = diag([1/M(1,1);1/M(2,2);1/M(3,3);1/M(4,4);1/M(5,5);1/M(6,6)]);

y = invM*K*e;

end

== matlab function omnimorph_controller_FL/Control/wait ==
  data: u input; y output; t input
function y = fcn(u,t)

    if t<1.5
        y = [0;0;0;0;0;0];
    else
        y = u;
    end

end

== matlab function omnimorph_controller_FL/Attitude trajectory ==
  data: R_des output; omega output; omega_dt output; t input; config parameter
function [R_des,omega,omega_dt] = fcn(t,config)

% Rotation about an axis
if t<7
   R_des = Rz(0)*Ry(0)*Rx(0);
   omega = [0;0;0];
   omega_dt = [0;0;0];
elseif t>=7 && t<13
   R_des = Rz(0)*Ry(0)*Rx(t-7);
   omega = [1;0;0];
   omega_dt = [0;0;0];
else
   R_des = Rz(0)*Ry(0)*Rx(0);
   omega = [0;0;0];
   omega_dt = [0;0;0];
end

% Peg-in-hole task
% if t<2
%     R_des = Rz(0)*Ry(0)*Rx(0);
%     omega = [0;0;0];
%     omega_dt = [0;0;0];
% else
%     R_des = Rz(0)*Ry(pi/4)*Rx(0);
%     omega = [0;0;0];
%     omega_dt = [0;0;0];
% end

%if t<2
%    R_des = Rz(0)*Ry(0)*Rx(0);
%    omega = [0;0;0];
%    omega_dt = [0;0;0];
%else
%    R_des = Rz(0)*Ry(t-2)*Rx(0);
%    omega = [0;1;0];
%    omega_dt = [0;0;0];
%end


% Sliding task
%R_des = Rz(0)*Ry(0)*Rx(0);
%omega = [0;0;0];
%omega_dt = [0;0;0];

end
